simulink model "quad_iris_model"  (R2014b)
settings: Solver=ode45  StartTime=0.0  StopTime=30.0  RelTol=1e-3
settings Model: Creator=ghost  LastModifiedBy=ghost

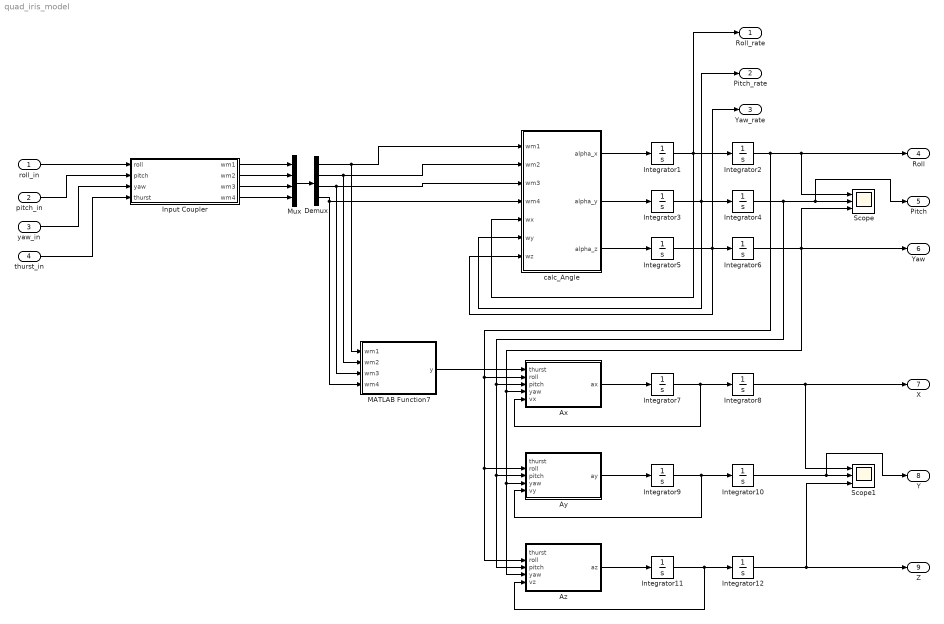
== system quad_iris_model ==
  roll_in : Inport
  pitch_in : Inport  Port=2
  yaw_in : Inport  Port=3
  thurst_in : Inport  Port=4
  Ax : MATLAB Function  TreatAsAtomicUnit=on
  Ay : MATLAB Function  TreatAsAtomicUnit=on
  Az : MATLAB Function  TreatAsAtomicUnit=on
  Demux : Demux
  Input Coupler : MATLAB Function  TreatAsAtomicUnit=on
  Integrator{1..12} (12 alike) : Integrator
  MATLAB Function7 : MATLAB Function  TreatAsAtomicUnit=on
  Mux : Mux
  Scope : Scope  NumInputPorts=3
      settings: YMin=-5~-5~-5  YMax=5~5~5
  Scope1 : Scope  NumInputPorts=3
      settings: YMin=-5~-5~-5  YMax=5~5~5
  calc_Angle : MATLAB Function  TreatAsAtomicUnit=on
  Roll_rate : Outport
  Pitch_rate : Outport  Port=2
  Yaw_rate : Outport  Port=3
  Roll : Outport  Port=4
  Pitch : Outport  Port=5
  Yaw : Outport  Port=6
  X : Outport  Port=7
  Y : Outport  Port=8
  Z : Outport  Port=9
  wires:
  calc_Angle/1(alpha_x) -> Integrator1/1
  calc_Angle/2(alpha_y) -> Integrator3/1
  calc_Angle/3(alpha_z) -> Integrator5/1
  MATLAB Function7/1(y) -> Ax/1(thurst)
  Integrator7/1 -> Ax/5(vx), Integrator8/1
  Az/1(az) -> Integrator11/1
  Integrator11/1 -> Az/5(vz), Integrator12/1
  Ay/1(ay) -> Integrator9/1
  Integrator9/1 -> Ay/5(vy), Integrator10/1
  Ax/1(ax) -> Integrator7/1
  Integrator10/1 -> Y/1, Scope1/2
  Integrator8/1 -> X/1, Scope1/1
  Integrator12/1 -> Z/1, Scope1/3
  Mux/1 -> Demux/1
  Demux/1 -> calc_Angle/1(wm1), MATLAB Function7/1(wm1)
  Demux/2 -> calc_Angle/2(wm2), MATLAB Function7/2(wm2)
  Demux/3 -> MATLAB Function7/3(wm3), calc_Angle/3(wm3)
  Demux/4 -> MATLAB Function7/4(wm4), calc_Angle/4(wm4)
  roll_in/1 -> Input Coupler/1(roll)
  pitch_in/1 -> Input Coupler/2(pitch)
  yaw_in/1 -> Input Coupler/3(yaw)
  thurst_in/1 -> Input Coupler/4(thurst)
  Input Coupler/1(wm1) -> Mux/1
  Input Coupler/2(wm2) -> Mux/2
  Input Coupler/3(wm3) -> Mux/3
  Input Coupler/4(wm4) -> Mux/4
  Integrator5/1 -> Yaw_rate/1, calc_Angle/7(wz), Integrator6/1
  Integrator1/1 -> Roll_rate/1, calc_Angle/5(wx), Integrator2/1
  Integrator3/1 -> Pitch_rate/1, Integrator4/1, calc_Angle/6(wy)
  Integrator6/1 -> Scope/3, Yaw/1, Az/4(yaw), Ay/4(yaw), Ax/4(yaw)
  Integrator4/1 -> Pitch/1, Scope/2, Ax/3(pitch), Az/3(pitch), Ay/3(pitch)
  Integrator2/1 -> Ax/2(roll), Ay/2(roll), Az/2(roll), Roll/1, Scope/1

== matlab function quad_iris_model/Input Coupler ==
  data: roll input; wm1 output; pitch input; yaw input; thurst input; wm2 output; wm3 output; wm4 output
function [wm1, wm2, wm3, wm4] = input_coupler(roll, pitch, yaw, thurst)
%#codegen

% 控制耦合
% 输入是归一化的，-1~1

% 基础输入 1000
thurst_bias = 1407;

% 去归一化
roll  = roll  * 500;
pitch = pitch * 500;
yaw   = yaw   * 500;
thurst = thurst * 1000;

wm1 = thurst + thurst_bias - roll - pitch + yaw;
wm2 = thurst + thurst_bias + roll + pitch + yaw;
wm3 = thurst + thurst_bias + roll - pitch - yaw;
wm4 = thurst + thurst_bias - roll + pitch - yaw;


return;

== matlab function quad_iris_model/MATLAB Function7 ==
  data: wm1 input; y output; wm2 input; wm3 input; wm4 input
function y = thurst(wm1, wm2, wm3, wm4)
%#codegen

k1 = 3.1 * 10^-7;
y = k1 * (wm1^2 + wm2^2 + wm3^2 + wm4^2);
return;

== matlab function quad_iris_model/Ax ==
  data: thurst input; roll input; pitch input; ax output; yaw input; vx input
function ax = calc_ax(thurst, roll, pitch, yaw, vx)
%#codegen
% roll  -> alpha
% pitch -> beta
% yaw   -> gamma

m  = 0.25;
g  = 9.81;
kf = 0;

ax = thurst * (sin(roll) * sin(yaw) + cos(roll) * sin(pitch) * cos(yaw));
ax = ax - kf * vx;
ax = ax / m;

return;

== matlab function quad_iris_model/Ay ==
  data: thurst input; roll input; pitch input; ay output; yaw input; vy input
function ay = calc_ay(thurst, roll, pitch, yaw, vy)
%#codegen
% roll  -> alpha
% pitch -> beta
% yaw   -> gamma

m  = 0.25;
g  = 9.81;
kf = 0;

ay = thurst * (-sin(roll) * cos(yaw) + cos(roll) * sin(pitch) * sin(yaw));
ay = ay - kf * vy;
ay = ay / m;

return;

== matlab function quad_iris_model/Az ==
  data: thurst input; roll input; pitch input; az output; yaw input; vz input
function az = calc_az(thurst, roll, pitch, yaw, vz)
%#codegen
% roll  -> alpha
% pitch -> beta
% yaw   -> gamma

m  = 0.25;
g  = 9.81;
kf = 0;

az = thurst * (cos(roll) * cos(pitch));
az = az / m - g;

return;

== matlab function quad_iris_model/calc_Angle ==
  data: wm1 input; wm2 input; wm3 input; wm4 input; alpha_x output; alpha_y output; alpha_z output; wx input; wy input; wz input
function [alpha_x, alpha_y, alpha_z] = calc_alpha(wm1,wm2, wm3, wm4, wx, wy, wz)
%#codegen

lf = 0.25;
lr = 0.28;
yakee = 60 * pi / 180;
zulu  = 25 * pi / 180;

Jx = 0.033;
Jy = 0.042;
Jz = 0.061;

m  = 0.25;
g  = 9.81;
kf = 0;

kt = 3.10 * 10^-7;
kq = 1.12 * 10^-6;

Mx = kt * ((wm2^2 - wm4^2) * sin(zulu) * lr + (wm3^2 - wm1^2)  * sin(yakee) * lf);
My = kt * ((wm2^2 + wm4^2) * cos(zulu) * lr + (-wm3^2 - wm1^2) * cos(yakee) * lf);
Mz = kq * ((wm2^2 - wm4^2) * lr + (wm1^2 - wm3^2) * lf);

alpha_x = Mx + (Jy - Jz) * wy * wz;
alpha_x = alpha_x / Jx;

alpha_y = My + (Jz - Jx) * wz * wx;
alpha_y = alpha_y / Jy;

alpha_z = Mz + (Jx - Jy) * wx * wy;
alpha_z = alpha_z / Jz;


return;
